simulink subsystem "elastic_buffer"  (R2022b)
settings: Solver=VariableStepAuto  StartTime=0.0  StopTime=10.0  RelTol=1e-3
settings Model: Creator=Ali-Laptop  LastModifiedBy=Ali-Laptop

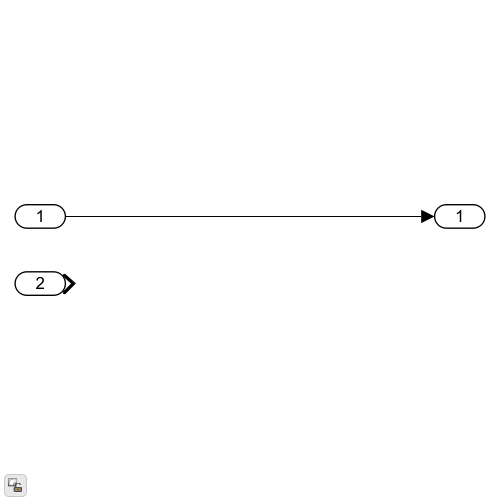
[thumbnail: Simulink's stored preview of the top-level diagram]
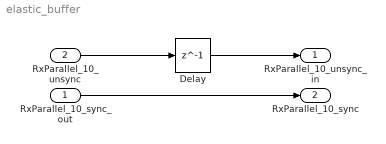
== system elastic_buffer ==
  RxParallel_10_sync_out : Inport
  RxParallel_10_unsync : Inport  Port=2
  Delay : Delay  DelayLength=1
  RxParallel_10_unsync_in : Outport
  RxParallel_10_sync : Outport  Port=2
  wires:
  RxParallel_10_unsync/1 -> Delay/1
  RxParallel_10_sync_out/1 -> RxParallel_10_sync/1
  Delay/1 -> RxParallel_10_unsync_in/1
